simulink model "vkr_zagr"  (R2023b)
settings: Solver=ode5  StartTime=0  StopTime=500  FixedStep=0.1  RelTol=1e-3
libraries: slpidlib x2
settings Model: Creator=Анастасия  LastModifiedBy=Анастасия

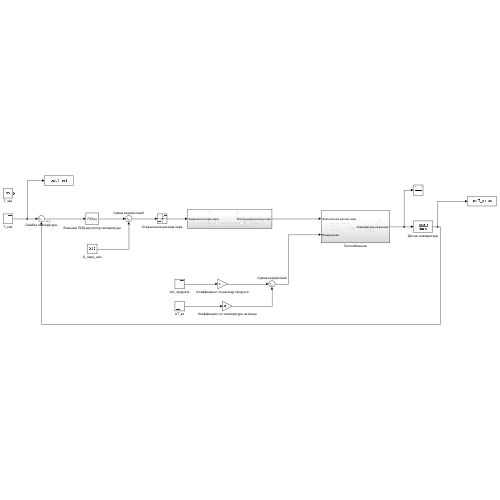
[thumbnail: Simulink's stored preview of the top-level diagram]
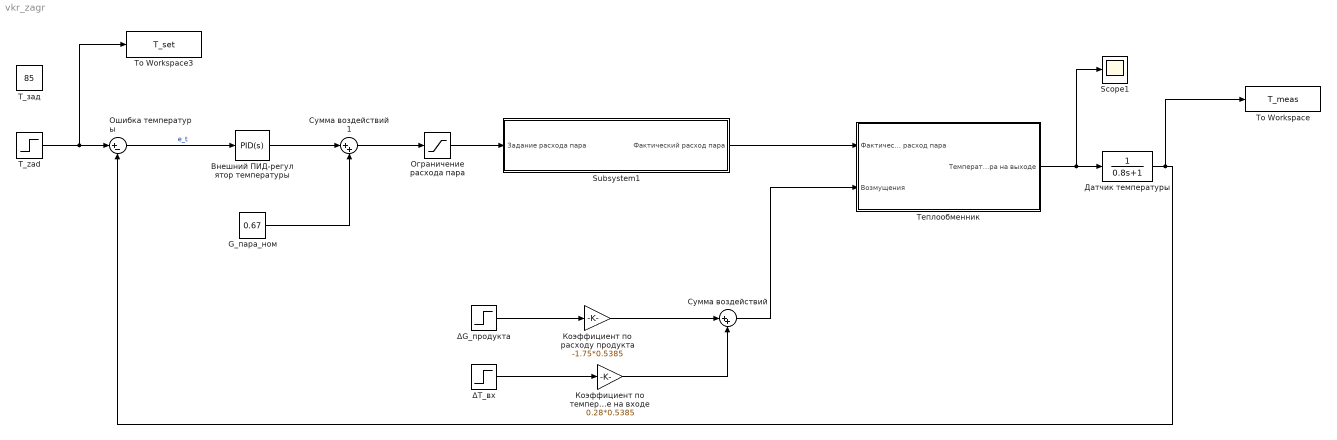
== system vkr_zagr ==
  G_пара_ном : Constant  Value=0.67
  Scope1 : Scope
  Subsystem1 : Subsystem
  T_zad : Step  Time=300  Before=85  After=90  SampleTime=0
  T_зад : Constant  Value=85
  To Workspace : ToWorkspace  VariableName=T_meas  SaveFormat=Timeseries  SampleTime=-1
  To Workspace3 : ToWorkspace  VariableName=T_set  SaveFormat=Structure With Time  SampleTime=-1
  ΔG_продукта : Step  Time=300  After=0  SampleTime=0
  ΔT_вх : Step  Time=300  After=0  SampleTime=0
  Внешний ПИД-регулятор температуры : slpidlib/PID Controller  Controller=PID  Form=Parallel  TimeDomain=Continuous-time  UseExternalTs=off  SampleTime=-1  IntegratorMethod=Forward Euler  FilterMethod=Forward Euler  ControllerParametersSource=internal  P=0.016  I=0.0004  UseKiTs=off  D=0.04  N=0.056  UseFilter=on  TunerSelectOption=Transfer Function Based (PID Tuner App)  InitialConditionSource=internal  InitialConditionForIntegrator=0  InitialConditionForFilter=0  DifferentiatorICPrevScaledInput=0  ExternalReset=none  TrackingMode=off  Kt=1  LimitOutput=off  SatLimitsSource=internal  UpperSaturationLimit=inf  LowerSaturationLimit=-inf  LinearizeAsGain=on  AntiWindupMode=none  Kb=1  LimitIntegrator=off  UpperIntegratorSaturationLimit=inf  LowerIntegratorSaturationLimit=-inf  POutMin=[]  POutMax=[]  IOutMin=[]  IOutMax=[]  DOutMin=[]  DOutMax=[]  NOutMin=[]  NOutMax=[]  SumOutMin=[]  SumOutMax=[]  SaturationOutMin=[]  SaturationOutMax=[]  PParamMin=[]  PParamMax=[]  IParamMin=[]  IParamMax=[]  DParamMin=[]  DParamMax=[]  NParamMin=[]  NParamMax=[]  KbParamMin=[]  KbParamMax=[]  KtParamMin=[]  KtParamMax=[]  KbOutMin=[]  KbOutMax=[]  KtOutMin=[]  KtOutMax=[]  IntegratorOutMin=[]  IntegratorOutMax=[]  FilterOutMin=[]  FilterOutMax=[]  SumI1OutMin=[]  SumI1OutMax=[]  SumI2OutMin=[]  SumI2OutMax=[]  SumI3OutMin=[]  SumI3OutMax=[]  SumI4OutMin=[]  SumI4OutMax=[]  SumDOutMin=[]  SumDOutMax=[]  DifferentiatorOutMin=[]  DifferentiatorOutMax=[]  FilterDiffOutCoefMin=[]  FilterDiffOutCoefMax=[]  ReciprocalOutMin=[]  ReciprocalOutMax=[]  SumDenOutMin=[]  SumDenOutMax=[]  SumNumOutMin=[]  SumNumOutMax=[]  DivideOutMin=[]  DivideOutMax=[]  UdiffTsProdOutMin=[]  UdiffTsProdOutMax=[]  NTsProdOutMin=[]  NTsProdOutMax=[]  UintegralTsProdOutMin=[]  UintegralTsProdOutMax=[]  UngainTsProdOutMin=[]  UngainTsProdOutMax=[]  ClampingZeroOutDataTypeStr=Inherit: Inherit via back propagation  ClampingZeroOutMin=[]  ClampingZeroOutMax=[]  FilterDenConstantOutDataTypeStr=Inherit: Inherit via back propagation  FilterDenConstantOutMin=[]  FilterDenConstantOutMax=[]  PCopyOutDataTypeStr=Inherit: Inherit via back propagation  PCopyOutMin=[]  PCopyOutMax=[]  NCopyOutDataTypeStr=Inherit: Inherit via back propagation  NCopyOutMin=[]  NCopyOutMax=[]  IntegratorContinuousStateAttributes=''  IntegratorStateMustResolveToSignalObject=off  IntegratorRTWStateStorageClass=Auto  FilterContinuousStateAttributes=''  FilterStateMustResolveToSignalObject=off  FilterRTWStateStorageClass=Auto  ParallelPVariant=InternalParameters  IdealPVariant=Disabled  IVariant=InternalParameters  DVariant=InternalParameters  IntegratorVariant=Continuous  SatVariant=Disabled  AWVariant=Passthrough  PCopyVariant=Disabled  TRVariant=Disabled  FdbkBlocksVariant=Forward  IdealPFdbkVariant=Disabled  SatFdbkVariant=Disabled  DerivativeFilterVariant=ContFilter  NVariant=InternalParameters  NCopyVariant=Disabled  FilterICVariant=InternalICsFilter  IntegratorICVariant=InternalICs  ExternalResetVariant=Disabled  TRSumVariant=Passthrough  SumFdbkVariant=Disabled  SumVariant=Sum_PID  TsampFilterVariant=InternalTs  TsampNgainVariant=Passthrough  TsampIntegralVariant=Disabled_SignalSpec  ExternalSaturationOutDataTypeStr=Inherit: Same as second input
  Датчик температуры : TransferFcn  Denominator=[0.8 1]
  Коэффициент по расходу продукта : Gain  Gain=-1.75*0.5385
  Коэффициент по температуре на входе : Gain  Gain=0.28*0.5385
  Ограничение расхода пара : Saturate  UpperLimit=1.5  LowerLimit=0
  Ошибка температуры : Sum  Inputs=|+-
  Сумма воздействий : Sum  Inputs=|++
  Сумма воздействий1 : Sum  Inputs=|++
  Теплообменник : Subsystem
  wires:
  Сумма воздействий1/1 -> Ограничение расхода пара/1
  Сумма воздействий/1 -> Теплообменник/2(Возмущения)
  Subsystem1/1(Фактический расход пара) -> Теплообменник/1(Фактический расход пара)
  G_пара_ном/1 -> Сумма воздействий1/2
  Датчик температуры/1 -> To Workspace/1, Ошибка температуры/2
  Ошибка температуры/1 -> Внешний ПИД-регулятор температуры/1  "e_t"
  ΔT_вх/1 -> Коэффициент по температуре на входе/1
  Коэффициент по температуре на входе/1 -> Сумма воздействий/2
  Коэффициент по расходу продукта/1 -> Сумма воздействий/1
  Ограничение расхода пара/1 -> Subsystem1/1(Задание расхода пара)
  Внешний ПИД-регулятор температуры/1 -> Сумма воздействий1/1
  ΔG_продукта/1 -> Коэффициент по расходу продукта/1
  Теплообменник/1(Температура на выходе) -> Scope1/1, Датчик температуры/1
  T_zad/1 -> To Workspace3/1, Ошибка температуры/1

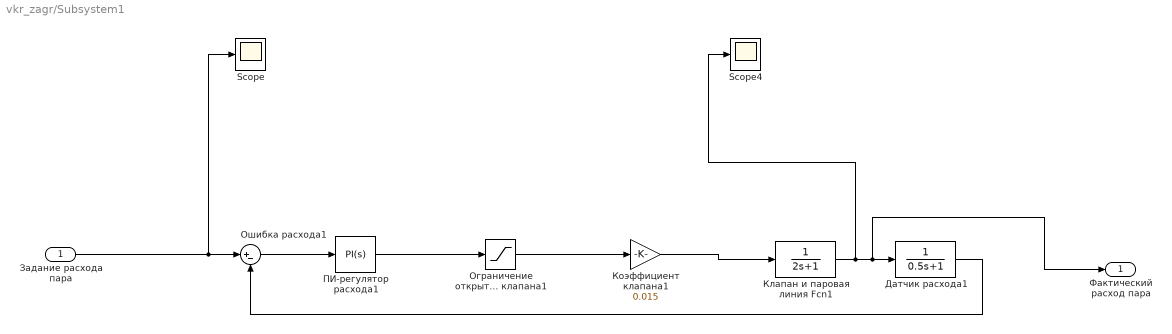
== system vkr_zagr/Subsystem1 ==
  Задание расхода пара : Inport
  Scope : Scope
  Scope4 : Scope
  Датчик расхода1 : TransferFcn  Denominator=[0.5,1]
  Клапан и паровая линия Fcn1 : TransferFcn  Denominator=[2 1]
  Коэффициент клапана1 : Gain  Gain=0.015
  Ограничение открытия клапана1 : Saturate  UpperLimit=100  LowerLimit=0
  Ошибка расхода1 : Sum  Inputs=|+-
  ПИ-регулятор расхода1 : slpidlib/PID Controller  Controller=PI  Form=Parallel  TimeDomain=Continuous-time  UseExternalTs=off  SampleTime=-1  IntegratorMethod=Forward Euler  FilterMethod=Forward Euler  ControllerParametersSource=internal  P=40  I=30  UseKiTs=off  D=0  N=100  UseFilter=on  TunerSelectOption=Transfer Function Based (PID Tuner App)  InitialConditionSource=internal  InitialConditionForIntegrator=0  InitialConditionForFilter=0  DifferentiatorICPrevScaledInput=0  ExternalReset=none  TrackingMode=off  Kt=1  LimitOutput=off  SatLimitsSource=internal  UpperSaturationLimit=inf  LowerSaturationLimit=-inf  LinearizeAsGain=on  AntiWindupMode=none  Kb=1  LimitIntegrator=off  UpperIntegratorSaturationLimit=inf  LowerIntegratorSaturationLimit=-inf  POutMin=[]  POutMax=[]  IOutMin=[]  IOutMax=[]  DOutMin=[]  DOutMax=[]  NOutMin=[]  NOutMax=[]  SumOutMin=[]  SumOutMax=[]  SaturationOutMin=[]  SaturationOutMax=[]  PParamMin=[]  PParamMax=[]  IParamMin=[]  IParamMax=[]  DParamMin=[]  DParamMax=[]  NParamMin=[]  NParamMax=[]  KbParamMin=[]  KbParamMax=[]  KtParamMin=[]  KtParamMax=[]  KbOutMin=[]  KbOutMax=[]  KtOutMin=[]  KtOutMax=[]  IntegratorOutMin=[]  IntegratorOutMax=[]  FilterOutMin=[]  FilterOutMax=[]  SumI1OutMin=[]  SumI1OutMax=[]  SumI2OutMin=[]  SumI2OutMax=[]  SumI3OutMin=[]  SumI3OutMax=[]  SumI4OutMin=[]  SumI4OutMax=[]  SumDOutMin=[]  SumDOutMax=[]  DifferentiatorOutMin=[]  DifferentiatorOutMax=[]  FilterDiffOutCoefMin=[]  FilterDiffOutCoefMax=[]  ReciprocalOutMin=[]  ReciprocalOutMax=[]  SumDenOutMin=[]  SumDenOutMax=[]  SumNumOutMin=[]  SumNumOutMax=[]  DivideOutMin=[]  DivideOutMax=[]  UdiffTsProdOutMin=[]  UdiffTsProdOutMax=[]  NTsProdOutMin=[]  NTsProdOutMax=[]  UintegralTsProdOutMin=[]  UintegralTsProdOutMax=[]  UngainTsProdOutMin=[]  UngainTsProdOutMax=[]  ClampingZeroOutDataTypeStr=Inherit: Inherit via back propagation  ClampingZeroOutMin=[]  ClampingZeroOutMax=[]  FilterDenConstantOutDataTypeStr=Inherit: Inherit via back propagation  FilterDenConstantOutMin=[]  FilterDenConstantOutMax=[]  PCopyOutDataTypeStr=Inherit: Inherit via back propagation  PCopyOutMin=[]  PCopyOutMax=[]  NCopyOutDataTypeStr=Inherit: Inherit via back propagation  NCopyOutMin=[]  NCopyOutMax=[]  IntegratorContinuousStateAttributes=''  IntegratorStateMustResolveToSignalObject=off  IntegratorRTWStateStorageClass=Auto  FilterContinuousStateAttributes=''  FilterStateMustResolveToSignalObject=off  FilterRTWStateStorageClass=Auto  ParallelPVariant=InternalParameters  IdealPVariant=Disabled  IVariant=InternalParameters  DVariant=Disabled  IntegratorVariant=Continuous  SatVariant=Disabled  AWVariant=Passthrough  PCopyVariant=Disabled  TRVariant=Disabled  FdbkBlocksVariant=Forward  IdealPFdbkVariant=Disabled  SatFdbkVariant=Disabled  DerivativeFilterVariant=Disabled  NVariant=Disabled  NCopyVariant=Disabled_SignalSpec  FilterICVariant=Disabled  IntegratorICVariant=InternalICs  ExternalResetVariant=Disabled  TRSumVariant=Passthrough  SumFdbkVariant=Disabled  SumVariant=Sum_PI  TsampFilterVariant=InternalTs  TsampNgainVariant=Passthrough  TsampIntegralVariant=Disabled_SignalSpec  ExternalSaturationOutDataTypeStr=Inherit: Same as second input
  Фактический расход пара : Outport
  wires:
  Клапан и паровая линия Fcn1/1 -> Scope4/1, Фактический расход пара/1, Датчик расхода1/1
  Коэффициент клапана1/1 -> Клапан и паровая линия Fcn1/1
  Ошибка расхода1/1 -> ПИ-регулятор расхода1/1
  ПИ-регулятор расхода1/1 -> Ограничение открытия клапана1/1
  Задание расхода пара/1 -> Scope/1, Ошибка расхода1/1
  Датчик расхода1/1 -> Ошибка расхода1/2
  Ограничение открытия клапана1/1 -> Коэффициент клапана1/1

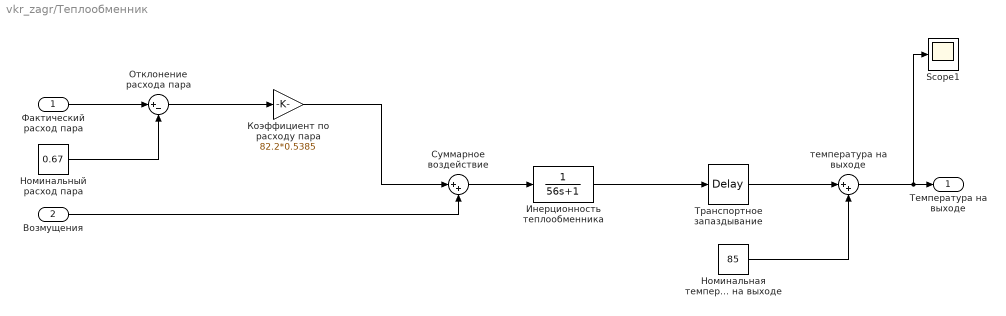
== system vkr_zagr/Теплообменник ==
  Фактический расход пара : Inport
  Возмущения : Inport  Port=2
  Scope1 : Scope
  Инерционность теплообменника : TransferFcn  Denominator=[56 1]
  Коэффициент по расходу пара : Gain  Gain=82.2*0.5385
  Номинальная температура на выходе : Constant  Value=85
  Номинальный расход пара : Constant  Value=0.67
  Отклонение расхода пара : Sum  Inputs=|+-
  Суммарное воздействие : Sum  Inputs=|++
  Транспортное запаздывание : TransportDelay  DelayTime=10
  температура на выходе : Sum  Inputs=|++
  Температура на выходе : Outport
  wires:
  Фактический расход пара/1 -> Отклонение расхода пара/1
  Номинальный расход пара/1 -> Отклонение расхода пара/2
  Отклонение расхода пара/1 -> Коэффициент по расходу пара/1
  Возмущения/1 -> Суммарное воздействие/2
  Коэффициент по расходу пара/1 -> Суммарное воздействие/1
  Суммарное воздействие/1 -> Инерционность теплообменника/1
  Инерционность теплообменника/1 -> Транспортное запаздывание/1
  Транспортное запаздывание/1 -> температура на выходе/1
  Номинальная температура на выходе/1 -> температура на выходе/2
  температура на выходе/1 -> Scope1/1, Температура на выходе/1
